simulink subsystem "fi_splitter"  (R2021b)
settings: Solver=VariableStepAuto  StartTime=0.0  StopTime=10.0  RelTol=1e-3
model mask{in_bitwidth=60, out_bitwidth=10}
settings Model: Creator=torha  LastModifiedBy=torha
settings SolverCC: AlgebraicLoopSolver=TrustRegion
settings DebuggingCC: SFMachineParentedDataDiag=warning

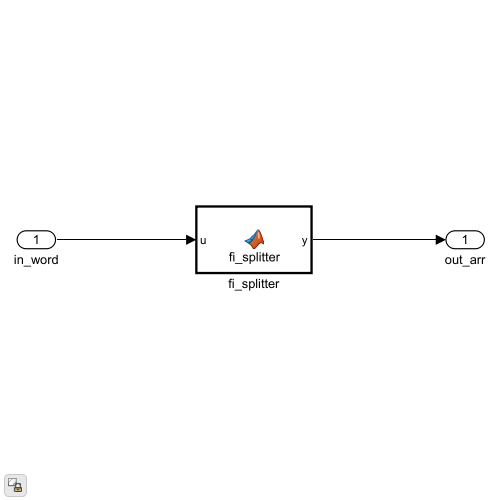
[thumbnail: Simulink's stored preview of the top-level diagram]
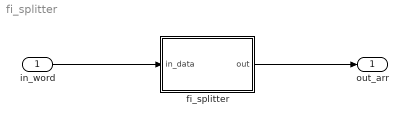
== system fi_splitter ==
  in_word : Inport
  fi_splitter : MATLAB Function  TreatAsAtomicUnit=on
  out_arr : Outport
  wires:
  fi_splitter/1(out) -> out_arr/1
  in_word/1 -> fi_splitter/1(in_data)

== matlab function fi_splitter/fi_splitter ==
  settings: fimath=fimath('RoundingMethod', 'Floor','OverflowAction', 'Wrap','ProductMode', 'FullPrecision', 'SumMode', 'FullPrecision')
  data: in_data input size=1; out output; out_bitwidth parameter size=1; in_bitwidth parameter size=1
function out = fi_splitter(in_data, out_bitwidth, in_bitwidth)
    in_data = castIntToFi(in_data);
    assert(isfi(in_data) && isfixed(in_data) && isscalar(in_data) && isreal(in_data));
    assert(in_data.WordLength == in_bitwidth);
    assert(~mod(in_bitwidth, out_bitwidth));
    out = zeros(1,in_bitwidth/out_bitwidth,'like',fi([],0,out_bitwidth,0));
    coder.unroll
    for k = 1:in_bitwidth/out_bitwidth
        out(in_bitwidth/out_bitwidth-k+1) = bitsliceget(in_data, k*out_bitwidth, (k-1)*out_bitwidth+1);
    end
end
